simulink model "baseline_super"  (R2021a)
settings: Solver=FixedStepAuto  StartTime=0.0  StopTime=10.0  FixedStep=framePeriod_s  RelTol=1e-3
undefined symbols (not defined in the file): Aircraft, framePeriod_s
libraries: simulink x30, pid_lib x11
(part 3 of 3)

== system baseline_super/WAYPOINT CONTROLLER/WP_NAV/heading_controller/heading_controller ==
  heading_cmd_rad : Inport
  <heading_rad> : Inport  Port=2
  D_heading : Constant  Value=Aircraft.Control.D_heading  OutDataTypeStr=single
  I_heading : Constant  Value=Aircraft.Control.I_heading  OutDataTypeStr=single
  PID Controller2 : pid_lib/PID Controller  Controller=PID  Form=Parallel  TimeDomain=Discrete-time  UseExternalTs=off  SampleTime=framePeriod_s  IntegratorMethod=Forward Euler  FilterMethod=Forward Euler  ControllerParametersSource=external  P=1.85  I=0.01  D=0  UseFilter=off  N=100  TunerSelectOption=Transfer Function Based (PID Tuner App)  InitialConditionSource=internal  InitialConditionForIntegrator=0  InitialConditionForFilter=0  DifferentiatorICPrevScaledInput=0  ExternalReset=none  TrackingMode=off  Kt=1  LimitOutput=on  SatLimitsSource=internal  UpperSaturationLimit=inf  LowerSaturationLimit=-inf  LinearizeAsGain=on  AntiWindupMode=clamping  Kb=2  POutMin=[]  POutMax=[]  IOutMin=[]  IOutMax=[]  DOutMin=[]  DOutMax=[]  NOutMin=[]  NOutMax=[]  SumOutMin=[]  SumOutMax=[]  SaturationOutMin=[]  SaturationOutMax=[]  PParamMin=[]  PParamMax=[]  IParamMin=[]  IParamMax=[]  DParamMin=[]  DParamMax=[]  NParamMin=[]  NParamMax=[]  KbParamMin=[]  KbParamMax=[]  KtParamMin=[]  KtParamMax=[]  KbOutMin=[]  KbOutMax=[]  KtOutMin=[]  KtOutMax=[]  IntegratorOutMin=[]  IntegratorOutMax=[]  FilterOutMin=[]  FilterOutMax=[]  SumI1OutMin=[]  SumI1OutMax=[]  SumI2OutMin=[]  SumI2OutMax=[]  SumI3OutMin=[]  SumI3OutMax=[]  SumI4OutMin=[]  SumI4OutMax=[]  SumDOutMin=[]  SumDOutMax=[]  DifferentiatorOutMin=[]  DifferentiatorOutMax=[]  FilterDiffOutCoefMin=[]  FilterDiffOutCoefMax=[]  ReciprocalOutMin=[]  ReciprocalOutMax=[]  SumDenOutMin=[]  SumDenOutMax=[]  SumNumOutMin=[]  SumNumOutMax=[]  DivideOutMin=[]  DivideOutMax=[]  UdiffTsProdOutMin=[]  UdiffTsProdOutMax=[]  NTsProdOutMin=[]  NTsProdOutMax=[]  UintegralTsProdOutMin=[]  UintegralTsProdOutMax=[]  UngainTsProdOutMin=[]  UngainTsProdOutMax=[]  IntegratorContinuousStateAttributes=''  IntegratorStateMustResolveToSignalObject=off  IntegratorRTWStateStorageClass=Auto  FilterContinuousStateAttributes=''  FilterStateMustResolveToSignalObject=off  FilterRTWStateStorageClass=Auto  ParallelPVariant=ExternalParameters  IdealPVariant=Disabled  IVariant=ExternalParameters  DVariant=ExternalParameters  IntegratorVariant=Discrete  SatVariant=Enabled  AWVariant=DiscClampingParallel  PCopyVariant=Disabled  TRVariant=Disabled  FdbkBlocksVariant=Forward  IdealPFdbkVariant=Disabled  SatFdbkVariant=Disabled  DerivativeFilterVariant=Differentiator  NVariant=Passthrough  NCopyVariant=Disabled_SignalSpec  FilterICVariant=InternalICsDifferentiator  IntegratorICVariant=InternalICs  ExternalResetVariant=Disabled  TRSumVariant=Passthrough  SumFdbkVariant=Disabled  SumVariant=Sum_PID  TsampFilterVariant=InternalTs  TsampNgainVariant=Passthrough  TsampIntegralVariant=Passthrough  ExternalSaturationOutDataTypeStr=Inherit: Same as second input
  P_heading : Constant  Value=Aircraft.Control.P_heading  OutDataTypeStr=single
  Saturation : Saturate  UpperLimit=Aircraft.Control.yaw_rate_max  LowerLimit=-Aircraft.Control.yaw_rate_max
  heading_error : Subsystem
  yaw_rate_cmd : Outport
  wires:
  P_heading/1 -> PID Controller2/2
  heading_cmd_rad/1 -> heading_error/1(heading_cmd_rad)
  I_heading/1 -> PID Controller2/3
  <heading_rad>/1 -> heading_error/2(heading_rad)
  PID Controller2/1 -> Saturation/1
  Saturation/1 -> yaw_rate_cmd/1
  heading_error/1(heading_error_rad) -> PID Controller2/1
  D_heading/1 -> PID Controller2/4

== system baseline_super/determine arm and mode selection/Failsafe_management/Battery failsafe/disarm motor ==
  Enable : EnablePort  StatesWhenEnabling=reset
  Compare To Constant2 : simulink/Logic and Bit Operations/Compare To Constant  relop=>  const=15  OutDataTypeStr=boolean
  Constant : Constant  Value=framePeriod_s
  Sum : Sum  Inputs=|++
  Unit Delay : UnitDelay  SampleTime=-1  HasFrameUpgradeWarning=on
  battery_low_trigger : Outport
  wires:
  Compare To Constant2/1 -> battery_low_trigger/1
  Sum/1 -> Compare To Constant2/1, Unit Delay/1
  Unit Delay/1 -> Sum/2
  Constant/1 -> Sum/1

== system baseline_super/WAYPOINT CONTROLLER/WP_NAV/Horizontal position controller/Horizontal_position_controller/convert to ve_cmd ==
  speed_cmd_mps : Inport
  bearing_to_target_rad : Inport  Port=2
  Cos : Trigonometry  Operator=cos
  Product : Product
  Product1 : Product
  Sin : Trigonometry
  ve_x_cmd : Outport
  ve_y_cmd : Outport  Port=2
  wires:
  Product/1 -> ve_x_cmd/1
  speed_cmd_mps/1 -> Product/1, Product1/1
  bearing_to_target_rad/1 -> Cos/1, Sin/1
  Cos/1 -> Product/2
  Sin/1 -> Product1/2
  Product1/1 -> ve_y_cmd/1

== system baseline_super/WAYPOINT CONTROLLER/WP_NAV/Horizontal position controller/Horizontal_position_controller/inertial_to_body conversion ==
  ve_xy : Inport
  heading_rad : Inport  Port=2
  2D rotation from NED_xy to body_xy : Subsystem
  Demux : Demux  Outputs=2
  Product : Product  Multiplication=Matrix(*)
  vb_x : Outport
  vb_y : Outport  Port=2
  wires:
  Demux/1 -> vb_x/1  "vb_x"
  Product/1 -> Demux/1  "vb_xy"
  heading_rad/1 -> 2D rotation from NED_xy to body_xy/1(<heading_rad>)
  ve_xy/1 -> Product/2
  2D rotation from NED_xy to body_xy/1(2D_rot) -> Product/1
  Demux/2 -> vb_y/1  "vb_y"

== system baseline_super/WAYPOINT CONTROLLER/WP_NAV/heading_controller/heading_controller/heading_error ==
  heading_cmd_rad : Inport
  heading_rad : Inport  Port=2
  Abs : Abs
  Compare To Constant : simulink/Logic and Bit Operations/Compare To Constant  relop=>  const=pi  OutDataTypeStr=boolean
  Constant : Constant  Value=2*pi  OutDataTypeStr=single
  Product : Product
  Sign : Signum
  Subtract : Sum  Inputs=+-
  Subtract1 : Sum  Inputs=+-
  Switch : Switch  Criteria=u2 > Threshold
  heading_error_rad : Outport
  wires:
  heading_cmd_rad/1 -> Subtract/1
  heading_rad/1 -> Subtract/2
  Subtract/1 -> Abs/1, Switch/3, Subtract1/1, Sign/1
  Compare To Constant/1 -> Switch/2
  Subtract1/1 -> Switch/1
  Switch/1 -> heading_error_rad/1
  Abs/1 -> Compare To Constant/1
  Sign/1 -> Product/1
  Product/1 -> Subtract1/2
  Constant/1 -> Product/2

== system baseline_super/WAYPOINT CONTROLLER/WP_NAV/Horizontal position controller/Horizontal_position_controller/inertial_to_body conversion/2D rotation from NED_xy to body_xy ==
  <heading_rad> : Inport
  Cos : Trigonometry  Operator=cos
  Gain : Gain  Gain=-1
  Mux : Mux
  Reshape : Reshape  OutputDimensionality=Customize  OutputDimensions=[2,2]
  Sin : Trigonometry
  2D_rot : Outport
  wires:
  <heading_rad>/1 -> Sin/1, Cos/1
  Mux/1 -> Reshape/1
  Sin/1 -> Mux/3, Gain/1
  Cos/1 -> Mux/1, Mux/4
  Reshape/1 -> 2D_rot/1
  Gain/1 -> Mux/2

== matlab function baseline_super/determine arm and mode selection/determine submode/waypoint submodes/determine_target_pos ==
  data: fp_x input; target_pos output single size=3; fp_y input; fp_z input; home_lat_rad input; home_lon_rad input; home_alt input
function target_pos = determine_target_pos(fp_x, fp_y, fp_z, home_lat_rad, home_lon_rad, home_alt)


% target_pos = flight_plan_to_ned(flight_plan, cur_wp, home_lat_rad, home_lon_rad, home_alt);

target_pos = mission_item_to_ned(fp_x, fp_y, fp_z, home_lat_rad, home_lon_rad, home_alt);

end

== matlab function baseline_super/determine arm and mode selection/determine submode/waypoint submodes/determine_wp_submode ==
  data: autocontinue input; cmd input; sub_mode output int8; target_pos input; ned_pos input; cur_mode input; Aircraft_Control_wp_radius input size=1
function sub_mode = determine_wp_submode(autocontinue, cmd, target_pos, ned_pos, cur_mode, Aircraft_Control_wp_radius)

sub_mode = cur_mode;

if cmd == 20
    sub_mode = int8(3); % RTL
    
elseif cmd == 16
    diff = target_pos - ned_pos;
    reached_wp = norm(diff) <= Aircraft_Control_wp_radius;
    if cur_mode ~= 3 && reached_wp && ~autocontinue
        sub_mode = int8(1); % pos hold
    end
end

end

== matlab function baseline_super/determine arm and mode selection/determine submode/rtl submodes/determine_rtl_submode ==
  data: target_pos input; sub_mode output; ned_pos input; cur_mode input; Aircraft_Control_wp_radius input
function sub_mode = determine_rtl_submode(target_pos, ned_pos, cur_mode, Aircraft_Control_wp_radius)

sub_mode = cur_mode;
diff = target_pos - ned_pos;
if norm(diff) <= Aircraft_Control_wp_radius
    sub_mode = int8(4); % land
end

end

== matlab function baseline_super/WAYPOINT CONTROLLER/wp_completion_check/check_wp_reached ==
  data: target_pos input; reached output; ned_pos input; autocontinue input; Aircraft_Control_wp_radius input
function reached = check_wp_reached(target_pos, ned_pos, autocontinue, Aircraft_Control_wp_radius)

diff = target_pos - ned_pos;
reached = norm(diff) <= Aircraft_Control_wp_radius && autocontinue;

== matlab function baseline_super/WAYPOINT CONTROLLER/determine target/determine_target ==
  data: cur_target_pos_m input; cur_target_pos_m output size=3; prev_target_pos_m input; home_lat input; home_lon input; home_alt input; cur_target_heading_rad output single size=1; max_v_z_mps output single size=1; max_v_hor_mps output single size=1; Aircraft_Control_v_z_up_max input; Aircraft_Control_v_hor_max input
function [cur_target_pos_m, cur_target_heading_rad, max_v_z_mps, ...
          max_v_hor_mps] = determine_target(cur_target_pos_m, prev_target_pos_m, home_lat, ...
                                            home_lon, home_alt, ... ned_pos_m, ...
                                            Aircraft_Control_v_z_up_max, ...
                                            Aircraft_Control_v_hor_max)

% cur_target_pos_m = flight_plan_to_ned(flight_plan, cur_ind, home_lat, home_lon, home_alt);
% 
% prev_ind = cur_ind - 1;
% if prev_ind < 0
%     prev_target_pos_m = ned_pos_m;
% else
%     prev_target_pos_m = flight_plan_to_ned(flight_plan, prev_ind, home_lat, home_lon, home_alt);
% end

diff = cur_target_pos_m - prev_target_pos_m;

xy_mag = norm(diff(1:2));

cur_target_heading_rad = atan2(diff(2), diff(1));
max_v_z_mps = abs(-diff(3) * Aircraft_Control_v_hor_max / xy_mag);
max_v_hor_mps = abs(xy_mag * Aircraft_Control_v_z_up_max / -diff(3));

== matlab function baseline_super/WAYPOINT CONTROLLER/determine target/determine_current_tar_pos ==
  data: fp_x input; cur_target_pos output; fp_y input; fp_z input; home_lat_rad input; home_lon_rad input; home_alt input
function cur_target_pos = determine_current_tar_pos(fp_x, fp_y, fp_z, ...
                                                    home_lat_rad, home_lon_rad, home_alt)

cur_target_pos = mission_item_to_ned(fp_x, fp_y, fp_z, home_lat_rad, home_lon_rad, home_alt);

end

== matlab function baseline_super/WAYPOINT CONTROLLER/determine target/calc_prev_target_pos/determine_prev_tar_pos ==
  data: fp_x input; pref_target_pos output; fp_y input; fp_z input; home_lat_rad input; home_lon_rad input; home_alt input
function pref_target_pos = determine_prev_tar_pos(fp_x, fp_y, fp_z, ...
                                                    home_lat_rad, home_lon_rad, home_alt)

pref_target_pos = mission_item_to_ned(fp_x, fp_y, fp_z, home_lat_rad, home_lon_rad, home_alt);

end
